simulink model "EngineDynamometer"  (R2025b)
settings: configuration reference "EngDynoVariable" (kept outside this file)
model workspace (MAT data in the model file):
  DynOperatingPts = timeseries
  DynOperatingPts.Name = 'Dynamic Operating Points'
  DynOperatingPts.DataInfo = tsdata.datametadata
  DynOperatingPts.DataInfo.Interpolation = tsdata.interpolation
  DynOperatingPts.DataInfo.Interpolation.Fhandle : function handle (value not decoded)
  DynOperatingPts.DataInfo.Interpolation.Name = 'linear'
  DynOperatingPts.TimeInfo = tsdata.timemetadata
  DynOperatingPts.TimeInfo.Length = 1281
  DynOperatingPts.TimeInfo.DuplicateTimes = 0
  DynOperatingPts.TimeInfo.Time_ = [0 0.001 7.75860549558 7.75960549558 8.75958684985 8.76058684985 10.7615495584 10.7625495584 11.7625309127 11.7635309127 13.7644936212 13.7654936212 ... (1281 elements, 1281x1)]
  DynOperatingPts.TimeInfo.Initialized = 1
  DynOperatingPts.QualityInfo = tsdata.qualmetadata
  DynOperatingPts.Data_ = [0 750 750 750 750 750 750 750 750 750 750 750 ... (2562 elements, 1281x2)]
undefined symbols (not defined in the file): CiDynoMaxTurboSpd, CiDynoSSSpdCmd, CiDynoSSTrqCmd, DynoResultsBlock, EnvAbsPrs, EnvAirTemp, EnvRair, ExhCamPhaseCmd, InjPw, IntkCamPhaseCmd, Line, PlntEngAfrStoich, PlntEngCps, PlntEngNCyl, PlntEngSinj, PlntEngVd, si, si0, SiDynoMaxTurboSpd, SiDynoOpenLoopEngSpdCmdPts, SiDynoOpenLoopExhCamPhsCmdPts, SiDynoOpenLoopIntCamPhsCmdPts, SiDynoOpenLoopLambdaCmdPts, SiDynoOpenLoopMaxMAP, SiDynoOpenLoopSpkDeltaCmdPts, SiDynoOpenLoopSteadyStateWaitLimit, SiDynoOpenLoopTpCmdPts, SiDynoOpenLoopWAPCmdPts, SiDynoSSSpdCmd, SiDynoSSTrqCmd, SiDynoSSWaitLim, SpkAdv, ThrPosPctCmd, WgAreaPctCmd
libraries: autolibutils x4, autolibpowerinfoutils x1, simulink x1
(part 1 of 3)
CloseFcn:
  | wkspvarnam = get_param(strcat(bdroot(gcb),'/Subsystem5'),'MbcTaskList');
  | clear(wkspvarnam)
  | clear wkspvarnam
settings Model: DataDictionary=VirtualDynoTemplate.sldd  ModifiedByFormat=The MathWorks, Inc.  SimulationMode=accelerator  PauseTimes=4395  NumberOfSteps=1000  SnapshotBufferSize=20  SnapshotInterval=1000  Creator=The MathWorks, Inc.  LastModifiedBy=The MathWorks, Inc.
settings ConfigSetRef: SourceName=EngDynoVariable

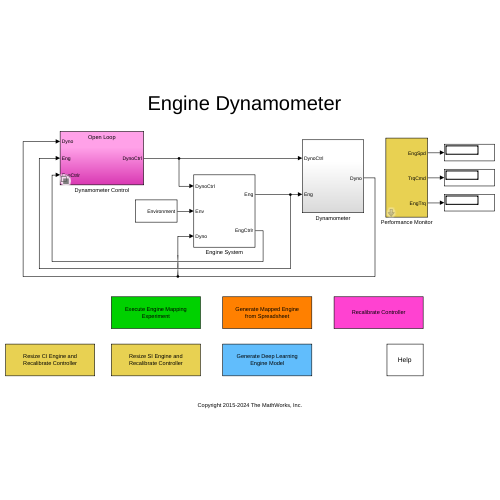
[thumbnail: Simulink's stored preview of the top-level diagram]
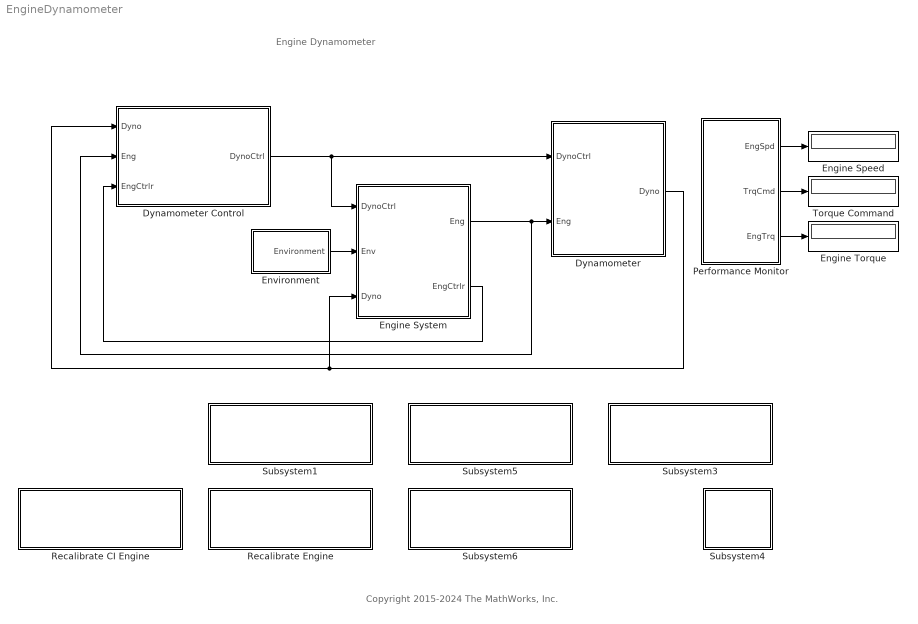
== system EngineDynamometer ==
  note: Engine Dynamometer
  note: Copyright 2015-2024 The MathWorks, Inc.
  Dynamometer : Subsystem
  Dynamometer Control : Subsystem  Variant=on  VariantControlMode=label  LabelModeActiveChoice=OpenLoop
  Engine Speed : Display
      settings: Decimation=100
  Engine System : Subsystem
      mask Display:
      | engplant = strcat(gcb,'/Engine Plant/Engine');
      | engvar = get_param(engplant,'ActiveVariant');
      | engvarp = strcat(engplant,'/',engvar);
      | istagged = false;
      | tagt = get_param(engvarp,'Tag');
      | if contains(engvar,'Mapped') && ~isempty(tagt)
      |     istagged = strcmp(tagt,'MappedEngCalByMBC');
      | end
      | ImageName = which('mbc_app_24.png');
      | if istagged
      |     if ~isempty(ImageName)
      |         IconImg = imread(ImageName,'png');
      |         MaskImg = 256*ones(150, 150,3);
      |         MaskImg = uint8(MaskImg);
      |         Xstart = 125;
      |         Ystart = 0;
      |         MaskImg((1:size(IconImg, 1))+Ystart, (1:size(IconImg, 2))+Xstart, 1:3) = IconImg;
      |         image(MaskImg);
      |     end
      |     disp('Mapped Engine\n Calibrated by\nMBC Toolbox')
      | end
  Engine Torque : Display
      settings: Decimation=100
  Environment : Subsystem
  Performance Monitor : Subsystem  StartFcn=DynoResultsBlock(gcb, 'StartFcn');  StopFcn=DynoResultsBlock(gcb, 'StopFcn');  mask(Performance Monitor){SteadyWsVarName=SteadyDynoSimOut, XVarPopup=Engine speed (rpm), YVarPopup=Torque command (N*m), ZVarPopup=Measured engine torque (N*m), DynWsVarName=DynamicDynoSimOut, DispAtEndCheckbox=on, UseSdiViewCheckbox=on, SdiRunName=Dynamometer Results, SdiViewFileName=DynoSDI_config.mldatx, ShowWaitbarCheckbox=on, NoPlot=si0}
      mask prompts: SteadyWsVarName "autoblks:autoblkDynoMask:wsVarName"; XVarPopup "autoblks:autoblkDynoMask:xAxisVar"; YVarPopup "autoblks:autoblkDynoMask:yAxisVar"; ZVarPopup "autoblks:autoblkDynoMask:zAxisVar"; DynWsVarName "autoblks:autoblkDynoMask:dynVarName"; DispAtEndCheckbox "autoblks:autoblkDynoMask:displayRes"; UseSdiViewCheckbox "autoblks:autoblkDynoMask:useSdiView"; SdiRunName "autoblks:autoblkDynoMask:sdiRunName"; SdiViewFileName "autoblks:autoblkDynoMask:sdiViewName"; ShowWaitbarCheckbox "autoblks:autoblkDynoMask:showWaitB"
      mask init:
      | DynoResultsBlock(gcb, 'Initialization');
      mask Help: helpview([docroot,'/toolbox/autoblks/helptargets.map'], 'siengine_dyno_refapp')
      mask TypeOptions XVarPopup: <EgrPct> | Air-fuel ratio | BSFC (g/(kW*hr)) | Compressor outlet temperature (C) | Compressor pressure ratio | EGR cooler outlet temperature (C) | EGR mass flow rate (g/s) | EGR valve area percent | EGR valve area percent command | Engine speed (rpm) | Engine speed command (rpm) | Estimated intake port mass flow rate (g/s) | Exhaust cam phase (degCrkRet) | Exhaust cam phase command (degCrkRet) | Exhaust manifold temperature (C) | Fuel mass flow rate (g/s) | Idle speed control torque command (N*m) | Injection pulse width (ms) | Intake cam phase (degCrkAdv) | Intake cam phase command (degCrkAdv) | Intake manifold pressure (kPa) | Intake manifold temperature (C) | Intake port mass flow rate (g/s) | Intercooler outlet temperature (C) | Load command | Measured engine torque (N*m) | Normalized air charge | Percent complete | Spark advance (degCrkAdv) | Steady state flag | Tailpipe CO emissions (g/s) | Tailpipe CO2 emissions (g/s) | Tailpipe HC emissions (g/s) | Tailpipe NOx emissions (g/s) | Throttle position percent | Throttle position percent command | Time (s) | Torque command (N*m) | Turbine outlet temperature (C) | Turbine pressure ratio | Turbocharger rack position | Turbocharger rack position command | Turbocharger shaft speed (rpm) | Wastegate area percent | Wastegate area percent command
      mask TypeOptions YVarPopup: None | <EgrPct> | Air-fuel ratio | BSFC (g/(kW*hr)) | Compressor outlet temperature (C) | Compressor pressure ratio | EGR cooler outlet temperature (C) | EGR mass flow rate (g/s) | EGR valve area percent | EGR valve area percent command | Engine speed (rpm) | Engine speed command (rpm) | Estimated intake port mass flow rate (g/s) | Exhaust cam phase (degCrkRet) | Exhaust cam phase command (degCrkRet) | Exhaust manifold temperature (C) | Fuel mass flow rate (g/s) | Idle speed control torque command (N*m) | Injection pulse width (ms) | Intake cam phase (degCrkAdv) | Intake cam phase command (degCrkAdv) | Intake manifold pressure (kPa) | Intake manifold temperature (C) | Intake port mass flow rate (g/s) | Intercooler outlet temperature (C) | Load command | Measured engine torque (N*m) | Normalized air charge | Percent complete | Spark advance (degCrkAdv) | Steady state flag | Tailpipe CO emissions (g/s) | Tailpipe CO2 emissions (g/s) | Tailpipe HC emissions (g/s) | Tailpipe NOx emissions (g/s) | Throttle position percent | Throttle position percent command | Time (s) | Torque command (N*m) | Turbine outlet temperature (C) | Turbine pressure ratio | Turbocharger rack position | Turbocharger rack position command | Turbocharger shaft speed (rpm) | Wastegate area percent | Wastegate area percent command
      mask TypeOptions ZVarPopup: None | <EgrPct> | Air-fuel ratio | BSFC (g/(kW*hr)) | Compressor outlet temperature (C) | Compressor pressure ratio | EGR cooler outlet temperature (C) | EGR mass flow rate (g/s) | EGR valve area percent | EGR valve area percent command | Engine speed (rpm) | Engine speed command (rpm) | Estimated intake port mass flow rate (g/s) | Exhaust cam phase (degCrkRet) | Exhaust cam phase command (degCrkRet) | Exhaust manifold temperature (C) | Fuel mass flow rate (g/s) | Idle speed control torque command (N*m) | Injection pulse width (ms) | Intake cam phase (degCrkAdv) | Intake cam phase command (degCrkAdv) | Intake manifold pressure (kPa) | Intake manifold temperature (C) | Intake port mass flow rate (g/s) | Intercooler outlet temperature (C) | Load command | Measured engine torque (N*m) | Normalized air charge | Percent complete | Spark advance (degCrkAdv) | Steady state flag | Tailpipe CO emissions (g/s) | Tailpipe CO2 emissions (g/s) | Tailpipe HC emissions (g/s) | Tailpipe NOx emissions (g/s) | Throttle position percent | Throttle position percent command | Time (s) | Torque command (N*m) | Turbine outlet temperature (C) | Turbine pressure ratio | Turbocharger rack position | Turbocharger rack position command | Turbocharger shaft speed (rpm) | Wastegate area percent | Wastegate area percent command
      mask DialogControl SteadyStateGroup Prompt: autoblks:autoblkDynoMask:steadySt
      mask DialogControl SteadyDesc Prompt: autoblks:autoblkDynoMask:steadyDesc
      mask DialogControl SteadyWsVarName Prompt: Steady state "To Workspace" variable name:
      mask DialogControl XVarPopup Prompt: X axis variable:
      mask DialogControl YVarPopup Prompt: Y axis variable:
      mask DialogControl ZVarPopup Prompt: Z axis variable:
      mask DialogControl PlotSteadyButton Prompt: autoblks:autoblkDynoMask:plotSS
      mask DialogControl PlotSteadyButton Callback: DynoResultsBlock(gcb, 'PlotSteadyButtonCallback');
      mask DialogControl DynamicGroup Prompt: autoblks:autoblkDynoMask:dynam
      mask DialogControl DynamicDesc Prompt: autoblks:autoblkDynoMask:plotDyn
      mask DialogControl DynWsVarName Prompt: Dynamic "To Workspace" variable name:
      mask DialogControl DispAtEndCheckbox Prompt: Display results at end of simulation
      mask DialogControl UseSdiViewCheckbox Prompt: Open Simulation Data Inspector view
      mask DialogControl SdiRunName Prompt: Simulation Data Inspector run name:
      mask DialogControl SdiViewFileName Prompt: Simulation Data Inspector view file name:
      mask DialogControl PlotDynamicButton Prompt: autoblks:autoblkDynoMask:plotDynButton
      mask DialogControl PlotDynamicButton Callback: DynoResultsBlock(gcb, 'PlotDynamicButtonCallback');
      mask DialogControl WaitbarGroup Prompt: autoblks:autoblkDynoMask:waitB
      mask DialogControl ShowWaitbarCheckbox Prompt: Show wait bar
  Recalibrate CI Engine : Subsystem  mask{EngReszSpecType=Displacement, EngReszMaxPwrDesIn=103.7766, EngReszDispDesIn=1.5, EngReszMaxPwrDes=109.307, EngReszNumCylDes=4, EngReszMaxPwr=103.7766, EngReszNumCyl=4, EngReszDisp=1.5, EngReszIdleSpd=500, EngReszMaxTqSpd=2750, EngReszMaxTq=273.6, EngReszBestFuelPwr=66, EngReszBestFuelSpd=2750, EngReszBestFuelTq=229.3, EngReszBestFuelBSFC=196.4, EngReszSpdMaxPwr=4000, EngReszTqMaxPwr=247.7, EngReszIntkManVol=2.86, EngReszExhManVol=0.7, EngReszMaxTurboSpd=237952.67, EngReszTurboRotInert=0.006, EngReszInjSlp=6.45}
      mask prompts: EngReszSpecType "Power or displacement"; EngReszMaxPwrDesIn "Desired maximum power [kW]:"; EngReszDispDesIn "Desired displacement [L]:"; EngReszMaxPwrDes "Desired maximum power [kW]:"; EngReszNumCylDes "Desired number of cylinders:"; EngReszMaxPwr "Maximum power [kW]:"; EngReszNumCyl "Number of cylinders:"; EngReszDisp "Engine displacement [L]:"; EngReszIdleSpd "Idle speed [rpm]:"; EngReszMaxTqSpd "Speed for maximum torque [rpm]:"; EngReszMaxTq "Maximum torque [Nm]:"; EngReszBestFuelPwr "Power for best fuel [kW]:"; EngReszBestFuelSpd "Speed for best fuel [rpm]:"; EngReszBestFuelTq "Torque for best fuel [Nm]:"; EngReszBestFuelBSFC "BSFC for best fuel [g/kWh]:"; EngReszSpdMaxPwr "Speed for maximum power [rpm]:"; EngReszTqMaxPwr "Torque for maximum power [Nm]:"; EngReszIntkManVol "Intake manifold volume [L]:"; EngReszExhManVol "Exhaust manifold volume [L]:"; EngReszMaxTurboSpd "Maximum turbo speed [rpm]:"; EngReszTurboRotInert "Turbo rotor inertia [kg*m^2]:"; EngReszInjSlp "Fuel injector slope [mg/ms]:"
      mask help: Resize engine plant and re-calibrate engine controller based on desired maximum power level or displacement, and number of cylinders
      settings: OpenFcn=|
      | block=[bdroot '/Recalibrate CI Engine'];
      | 
      | modelStatus = get_param(bdroot,'SimulationStatus');
      | 
      | if ~bdIsLibrary(bdroot) && strcmp(modelStatus,'stopped')
      |    autoicon('autolibciengresize',block,'open');
      |    open_system(block,'mask');
      | elseif ~bdIsLibrary(bdroot) && ~strcmp(modelStatus,'stopped')
      | else
      | end
      | 
      | clear modelStatus;
      | clear block;
      mask Help: eval('autoblkshelp(''pt_ci_resize'')');
      mask TypeOptions EngReszSpecType: Power | Displacement
      mask Callback EngReszSpecType: autoicon('autolibciengresize',gcb,'resizebasis');
      mask DialogControl DescGroupVar Prompt: Resize engine and recalibrate controller
      mask DialogControl DescTextVar Prompt: Resize engine plant and re-calibrate engine controller based on desired maximum power level or displacement, and number of cylinders
      mask DialogControl ResizeEngButton Prompt: Resize Engine
      mask DialogControl ResizeEngButton Callback: autoicon('autolibciengresize',gcb,'resize');
      mask DialogControl CurrEngDesign Prompt: Current Engine Design
      mask Display: disp(getString(message('autoblks:autoblkDynoMask:resizeCiLabel')))
  Recalibrate Engine : Subsystem  mask(Engine resize and recalibrate tool){EngReszSpecType=Displacement, EngReszMaxPwrDesIn=115.0917, EngReszDispDesIn=1.5, EngReszMaxPwrDes=115.0917, EngReszNumCylDes=4, EngReszArchEngine=Line, EngReszTurb=on, EngReszEgr=on, Thr2=off, TrqSpec=off, EngReszDesMaxTq=228, TrqSpdSpec=off, EngReszReqMaxTqSpd=2571, EngReszMaxPwr=115.0917, EngReszDisp=1.5, EngReszNumCyl=4, EngReszIdleSpd=750, EngReszMaxTqSpd=2571, EngReszMaxTq=228, EngReszBestFuelPwr=41.1, EngReszBestFuelSpd=2571, EngReszBestFuelTq=152.7, EngReszBestFuelBSFC=225.9, EngReszSpdMaxPwr=5000, EngReszTqMaxPwr=219.8, EngReszThrDiam=50, EngReszIntkManVol=2.86, EngReszExhManVol=1.6, EngReszCompOutVol=2.6, EngReszMaxTurboSpd=232000, EngReszTurboRotInert=0.016, EngReszInjSlp=6.45, EngCurrArch=Line, EngCurrTurb=on, EngCurrEGR=on, EngCurrThr2=off, EngCurrMaxTq=0, EngCurrMaxTqSpd=0}
      mask prompts: EngReszSpecType "autoblks:autoblkDynoMask:powerOrDispl"; EngReszMaxPwrDesIn "autoblks:autoblkDynoMask:desMaxPower"; EngReszDispDesIn "autoblks:autoblkDynoMask:desMaxDispl"; EngReszMaxPwrDes "autoblks:autoblkDynoMask:desMaxPower"; EngReszNumCylDes "autoblks:autoblkDynoMask:desNCyls"; EngReszArchEngine "autoblks:autoblkDynoMask:engArch"; EngReszTurb "autoblks:autoblkDynoMask:turbo"; EngReszEgr "autoblks:autoblkDynoMask:egr"; Thr2 "autoblks:autoblkDynoMask:twinInt"; TrqSpec "autoblks:autoblkDynoMask:maxTrq"; EngReszDesMaxTq "autoblks:autoblkDynoMask:desTrq"; TrqSpdSpec "autoblks:autoblkDynoMask:spdTrq"; EngReszReqMaxTqSpd "autoblks:autoblkDynoMask:desSpd"; EngReszMaxPwr "autoblks:autoblkDynoMask:maxPwr"; EngReszDisp "autoblks:autoblkDynoMask:engDispl"; EngReszNumCyl "autoblks:autoblkDynoMask:nCyls"; EngReszIdleSpd "autoblks:autoblkDynoMask:idleSpd"; EngReszMaxTqSpd "autoblks:autoblkDynoMask:trqSpd"; EngReszMaxTq "autoblks:autoblkDynoMask:actTrq"; EngReszBestFuelPwr "autoblks:autoblkDynoMask:bestFuel"; EngReszBestFuelSpd "autoblks:autoblkDynoMask:bestSpd"; EngReszBestFuelTq "autoblks:autoblkDynoMask:bestTrq"; EngReszBestFuelBSFC "autoblks:autoblkDynoMask:bestBSFC"; EngReszSpdMaxPwr "autoblks:autoblkDynoMask:maxPwrSpd"; EngReszTqMaxPwr "autoblks:autoblkDynoMask:trqPwr"; EngReszThrDiam "autoblks:autoblkDynoMask:thrDia"; EngReszIntkManVol "autoblks:autoblkDynoMask:intVol"; EngReszExhManVol "autoblks:autoblkDynoMask:exhVol"; EngReszCompOutVol "autoblks:autoblkDynoMask:cmpVol"; EngReszMaxTurboSpd "autoblks:autoblkDynoMask:turboSpd"; EngReszTurboRotInert "autoblks:autoblkDynoMask:tInertia"; EngReszInjSlp "autoblks:autoblkDynoMask:injFlow"; EngCurrArch "autoblks:autoblkDynoMask:engArch"; EngCurrTurb "autoblks:autoblkDynoMask:turbo"; EngCurrEGR "autoblks:autoblkDynoMask:egr"; EngCurrThr2 "autoblks:autoblkDynoMask:twinInt"; EngCurrMaxTq "autoblks:autoblkDynoMask:desTrq"; EngCurrMaxTqSpd "autoblks:autoblkDynoMask:desSpd"
      mask help: autoblks:autoblkDynoMask:descText
      mask init:
      | autoicon('autolibsiengresize',gcb,'updateEng');
      settings: OpenFcn=|
      | block=[bdroot '/Recalibrate Engine'];
      | 
      | modelStatus = get_param(bdroot,'SimulationStatus');
      | 
      | if ~bdIsLibrary(bdroot) && strcmp(modelStatus,'stopped')
      |    autoicon('autolibsiengresize',block,'open');
      |    open_system(block,'mask');
      | end
      | 
      | clear modelStatus;
      | clear block;
      mask Help: eval('autoblkshelp(''pt_si_resize'')');
      mask TypeOptions EngReszSpecType: autoblks:autoblkDynoMask:pOpt | autoblks:autoblkDynoMask:dOpt
      mask Callback EngReszSpecType:
      | if autoblkschecksimstopped(gcb)
      |     autoicon('autolibsiengresize',gcb,'resizebasis');
      |     maskObj = Simulink.Mask.get(gcb);
      |     if strcmp(maskObj.getParameter('EngReszSpecType').Value,getString(message('autoblks:autoblkDynoMask:pOpt')))
      |         maskObj.getParameter('TrqSpec').set('Visible','off');
      |         maskObj.getParameter('TrqSpdSpec').set('Visible','off');
      |         maskObj.getParameter('EngReszDesMaxTq').set('Visible','off');
      |         maskObj.getParameter('EngReszReqMaxTqSpd').set('Visible','off');
      |     else
      |         maskObj.getParameter('TrqSpec').set('Visible','on');
      |         maskObj.getParameter('TrqSpdSpec').set('Visible','on');
      |         if strcmp(maskObj.getParameter('TrqSpec').Value,'on')
      |             maskObj.getParameter('EngReszDesMaxTq').set('Visible','on');
      |         end
      |         if strcmp(maskObj.getParameter('TrqSpdSpec').Value,'on')
      |             maskObj.getParameter('EngReszReqMaxTqSpd').set('Visible','on');
      |         end
      |     end
      | end
      mask TypeOptions EngReszArchEngine: autoblks:autoblkDynoMask:iOpt | autoblks:autoblkDynoMask:vOpt
      mask Callback EngReszArchEngine:
      | if autoblkschecksimstopped(gcb)
      |     maskObj = Simulink.Mask.get(gcb);
      |     thr2box = maskObj.getParameter('Thr2');
      |     if strcmp(maskObj.getParameter('EngReszArchEngine').Value,getString(message('autoblks:autoblkDynoMask:vOpt'))) && ...
      |             strcmp(maskObj.getParameter('EngReszTurb').Value,'on')
      |         thr2box.set('Visible','on');
      |     else
      |         thr2box.set('Visible','off');
      |     end
      | end
      mask Callback EngReszTurb:
      | if autoblkschecksimstopped(gcb)
      |     maskObj = Simulink.Mask.get(gcb);
      |     thr2box = maskObj.getParameter('Thr2');
      |     if strcmp(maskObj.getParameter('EngReszTurb').Value,'on')
      |         maskObj.getParameter('EngReszCompOutVol').set('Visible','on');
      |         maskObj.getParameter('EngReszMaxTurboSpd').set('Visible','on');
      |         maskObj.getParameter('EngReszTurboRotInert').set('Visible','on');
      |         if strcmp(maskObj.getParameter('EngReszArchEngine').Value,getString(message('autoblks:autoblkDynoMask:vOpt'))) && ...
      |                 strcmp(thr2box.Visible,'off')
      |             thr2box.set('Visible','on');
      |         end
      |     else
      |         maskObj.getParameter('EngReszCompOutVol').set('Visible','off');
      |         maskObj.getParameter('EngReszMaxTurboSpd').set('Visible','off');
      |         maskObj.getParameter('EngReszTurboRotInert').set('Visible','off');
      |         if strcmp(maskObj.getParameter('EngReszArchEngine').Value,getString(message('autoblks:autoblkDynoMask:vOpt'))) && ...
      |                 strcmp(thr2box.Visible,'on')
      |             thr2box.set('Visible','off');
      |         end
      |     end
      | end
      mask Callback TrqSpec:
      | if autoblkschecksimstopped(gcb)
      |     autoicon('autolibsiengresize',gcb,'defTrq'); % Update with default calculated value
      |     maskObj = Simulink.Mask.get(gcb);
      |     maskTrq = get_param(gcb,'EngReszDesMaxTq'); % Need to get the value set from autoblkssiengresize in order to update
      |     if strcmp(maskObj.getParameter('TrqSpec').Value,'on')
      |         maskObj.getParameter('EngReszDesMaxTq').set('Visible','on');
      |         set_param(gcb,'EngReszDesMaxTq',maskTrq); % Need to set updated value in order to update
      |     else
      |         maskObj.getParameter('EngReszDesMaxTq').set('Visible','off');
      |     end
      | end
      mask Callback TrqSpdSpec:
      | if autoblkschecksimstopped(gcb)
      |     autoicon('autolibsiengresize',gcb,'defSpd'); % Populate with calculated default value
      |     maskObj = Simulink.Mask.get(gcb);
      |     maskSpd = get_param(gcb,'EngReszReqMaxTqSpd'); % Need to get the value set from autoblkssiengresize in order to update
      |     if strcmp(maskObj.getParameter('TrqSpdSpec').Value,'on')
      |         maskObj.getParameter('EngReszReqMaxTqSpd').set('Visible','on');
      |         set_param(gcb,'EngReszReqMaxTqSpd',maskSpd); % Need to set updated value in order to update
      |     else
      |         maskObj.getParameter('EngReszReqMaxTqSpd').set('Visible','off');
      |     end
      | end
      mask DialogControl Container4 Prompt: autoblks:autoblkDynoMask:design
      mask DialogControl EngReszSpecType Prompt: Resize option
      mask DialogControl EngReszMaxPwrDesIn Prompt: Desired maximum power, EngReszMaxPwrDes [kW]:
      mask DialogControl EngReszDispDesIn Prompt: Desired displacement, EngReszDispDesIn [L]:
      mask DialogControl EngReszMaxPwrDes Prompt: Desired maximum power, EngReszMaxPwrDes [kW]:
      mask DialogControl EngReszNumCylDes Prompt: Desired number of cylinders, EngReszNumCylDes [-]:
      mask DialogControl EngReszArchEngine Prompt: Architecture
      mask DialogControl EngReszTurb Prompt: Turbocharger
      mask DialogControl EngReszEgr Prompt: EGR
      mask DialogControl Thr2 Prompt: Twin Intake
      mask DialogControl TrqSpec Prompt: Specify maximum torque
      mask DialogControl EngReszDesMaxTq Prompt: EngReszDesMaxTq [Nm]:
      mask DialogControl TrqSpdSpec Prompt: Specify speed at maximum torque
      mask DialogControl EngReszReqMaxTqSpd Prompt: EngReszReqMaxTqSpd [rpm]:
      mask DialogControl ResizeEngButton Prompt: autoblks:autoblkDynoMask:resizeButton
      mask DialogControl ResizeEngButton Callback: autoicon('autolibsiengresize',gcb,'resize');
      mask DialogControl Container6 Prompt: autoblks:autoblkDynoMask:perfSpecs
      mask DialogControl CurrEngDesign Prompt: autoblks:autoblkDynoMask:currEng
      mask DialogControl EngReszMaxPwr Prompt: Maximum power [kW]:
      mask DialogControl EngReszDisp Prompt: Engine displacement [L]:
      mask DialogControl EngReszNumCyl Prompt: Number of cylinders:
      mask DialogControl EngReszIdleSpd Prompt: Idle speed [rpm]:
      mask DialogControl EngReszMaxTqSpd Prompt: Speed for maximum torque [rpm]:
      mask DialogControl EngReszMaxTq Prompt: Maximum torque [Nm]:
      mask DialogControl EngReszBestFuelPwr Prompt: Power for best fuel [kW]:
      mask DialogControl EngReszBestFuelSpd Prompt: Speed for best fuel [rpm]:
      mask DialogControl EngReszBestFuelTq Prompt: Torque for best fuel [Nm]:
      mask DialogControl EngReszBestFuelBSFC Prompt: BSFC for best fuel [g/kWh]:
      mask DialogControl EngReszSpdMaxPwr Prompt: Speed for maximum power [rpm]:
      mask DialogControl EngReszTqMaxPwr Prompt: Torque for maximum power [Nm]:
      mask DialogControl EngReszThrDiam Prompt: Throttle bore diameter [mm]:
      mask DialogControl EngReszIntkManVol Prompt: Intake manifold volume [L]:
      mask DialogControl EngReszExhManVol Prompt: Exhaust manifold volume [L]:
      mask DialogControl EngReszCompOutVol Prompt: Compressor out volume [L]:
      mask DialogControl EngReszMaxTurboSpd Prompt: Maximum turbo speed [rpm]:
      mask DialogControl EngReszTurboRotInert Prompt: Turbo rotor inertia [kg*m^2]:
      mask DialogControl EngReszInjSlp Prompt: Fuel injector slope [mg/ms]:
      mask DialogControl EngCurrArch Prompt: Architecture
      mask DialogControl EngCurrTurb Prompt: Turbocharger
      mask DialogControl EngCurrEGR Prompt: EGR
      mask DialogControl EngCurrThr2 Prompt: Twin Intake
      mask DialogControl EngCurrMaxTq Prompt: EngReszDesMaxTq [Nm]:
      mask DialogControl EngCurrMaxTqSpd Prompt: EngReszReqMaxTqSpd [rpm]:
      mask Display: disp(getString(message('autoblks:autoblkDynoMask:resizeSiLabel')))
  Subsystem1 : Subsystem
      settings: OpenFcn=DynamometerStart(gcb, 'SteadyState')
      mask Display: disp(getString(message('autoblks:autoblkDynoMask:engMapLabel')))
  Subsystem3 : Subsystem  mask{NoMsk=0}
      settings: OpenFcn=|
      | engblk=[bdroot,'/Engine System/Engine Plant/Engine'];
      | engvar=get_param(engblk,'ActiveVariant');
      | if strcmp(engvar,'CI Engine') || strcmp(engvar,'CI Mapped Engine')
      |   RecalibrateCIController(gcb, 'OpenFcn')
      | else
      |   RecalibrateSIController(gcb, 'OpenFcn')
      | end
      | clear engblk engvar
      mask Display: disp(getString(message('autoblks:autoblkDynoMask:recalibLabel')))
  Subsystem4 : Subsystem  mask{SiOrCi=si}
      settings: OpenFcn=|
      | if strcmp(get_param(gcb, 'SiOrCi'),'sih2')
      |   helpview([docroot,'/toolbox/autoblks/helptargets.map'], 'sih2engine_dyno_refapp')
      | elseif strcmp(get_param(gcb, 'SiOrCi'),'ci')
      |   helpview([docroot,'/toolbox/autoblks/helptargets.map'], 'ciengine_dyno_refapp')
      | else
      |   helpview([docroot,'/toolbox/autoblks/helptargets.map'], 'siengine_dyno_refapp')
      | end
      mask Display: disp(getString(message('autoblks:autoblkDynoMask:helpLabel')))
  Subsystem5 : Subsystem  LoadFcn=[~]=GenerateMappedEngineCalibrations(gcb, 'CheckMBCLicense');  mask(Create Mapped Engine from Spreadsheet){SpreadsheetFileName=SiEngineData.xlsx, MappedEngMdlRefName=SiMappedEngine, MbcTaskList=mbctasklist}
      mask prompts: SpreadsheetFileName "autoblks:autoblkDynoMask:mapSheetFile"; MappedEngMdlRefName "autoblks:autoblkDynoMask:mappedEng"; MbcTaskList "MBC Task List"
      mask help: autoblks:autoblkDynoMask:descSheet
      mask init:
      | GenerateMappedEngineCalibrations(gcb, 'Init');
      settings: OpenFcn=|
      | [~]=GenerateMappedEngineCalibrations(gcb, 'EnableCalToolButton');
      | open_system(gcb, 'mask')
      mask Help: helpview([docroot,'/toolbox/autoblks/helptargets.map'], 'siengine_dyno_mapped')
      mask DialogControl DescTextVar Prompt: autoblks:autoblkDynoMask:descSheet
      mask DialogControl MBCHyperlink Prompt: autoblks:autoblkDynoMask:reqOpt
      mask DialogControl MBCHyperlink Callback: helpview([docroot,'/toolbox/mbc/helptargets.map'], 'mbc_landing_page')
      mask DialogControl Container3 Prompt: autoblks:autoblkDynoMask:step1
      mask DialogControl SpreadsheetFileName Prompt: Spreadsheet file:
      mask DialogControl SpreadsheetFileNameSelect Prompt: autoblks:autoblkDynoMask:ellipsis
      mask DialogControl SpreadsheetFileNameSelect Callback: GenerateMappedEngineCalibrations(gcb, 'SpreadsheetFileNameSelect');
      mask DialogControl GenMappedEngCalButton Prompt: autoblks:autoblkDynoMask:engCal
      mask DialogControl GenMappedEngCalButton Callback: GenerateMappedEngineCalibrations(gcb, 'GenMappedEngCalButton');
      mask DialogControl OpenCalToolButton Prompt: autoblks:autoblkDynoMask:openCal
      mask DialogControl OpenCalToolButton Callback: GenerateMappedEngineCalibrations(gcb, 'OpenMBCFiles');
      mask DialogControl MappedEngMdlRefName Prompt: Mapped engine model reference name
      mask Display: disp(getString(message('autoblks:autoblkDynoMask:mapSpreadLabel')))
  Subsystem6 : Subsystem
      settings: OpenFcn=[~,~,~,~,~]=FitSiEngineDL(bdroot(gcb));
      mask Display: disp(getString(message('autoblks:autoblkDynoMask:genDLengLabel')))
  Torque Command : Display
      settings: Decimation=100
  wires:
  Engine System/2(EngCtrlr) -> Dynamometer Control/3(EngCtrlr)
  Dynamometer Control/1(DynoCtrl) -> Dynamometer/1(DynoCtrl), Engine System/1(DynoCtrl)
  Dynamometer/1(Dyno) -> Dynamometer Control/1(Dyno), Engine System/3(Dyno)
  Engine System/1(Eng) -> Dynamometer Control/2(Eng), Dynamometer/2(Eng)
  Environment/1(Environment) -> Engine System/2(Env)
  Performance Monitor/3(EngTrq) -> Engine Torque/1
  Performance Monitor/1(EngSpd) -> Engine Speed/1
  Performance Monitor/2(TrqCmd) -> Torque Command/1

== system EngineDynamometer/Dynamometer ==
  DynoCtrl : Inport
  Eng : Inport  Port=2
  Bus Creator : BusCreator  Inputs=2
  Bus Selector : BusSelector  OutputSignals=EngPlnt.EngTrq,EngPlnt.EngSpdOut
  Dynamometer Motor Controller : Subsystem
  Dynamometer Plant : Subsystem
  Bus Element Out1 : Outport  PortName=Dyno  Element=DynoPlnt
  Bus Element Out : Outport  PortName=Dyno  Element=DynoCtrl
  tag scope: DynoResults=global
  wires:
  Bus Creator/1 -> [DynoResults]
  Eng/1 -> Bus Selector/1, Dynamometer Plant/1(Eng), Dynamometer Motor Controller/1(EngPlnt)
  Dynamometer Plant/1(DynoPlnt) -> [DynoPlnt], Bus Element Out1/1, Dynamometer Motor Controller/3(DynoPlnt)
  Dynamometer Motor Controller/1(DynoMotorCtrl) -> Dynamometer Plant/4(DynoCtrl)
  [DynoPlnt] -> Bus Creator/2  "DynoPlnt"
  [DynoCtrl] -> Bus Creator/1  "DynoCtrl"
  DynoCtrl/1 -> Bus Element Out/1, [DynoCtrl], Dynamometer Motor Controller/2(DynoCtrl)
  Bus Selector/1 -> Dynamometer Plant/2(EngTrq)  "<EngTrq>"
  Bus Selector/2 -> Dynamometer Plant/3("EngSpd ")  "<EngSpdOut>"

== system EngineDynamometer/Dynamometer Control ==
  Dyno : Inport
  Eng : Inport  Port=2
  EngCtrlr : Inport  Port=3
  Calibrate Throttle and Wastegate : Subsystem  VariantControl=CalThrWg
  Calibration Controller : Subsystem  VariantControl=CalCtrl
  Dynamic : Subsystem  VariantControl=Dynamic
  Open Loop : Subsystem  VariantControl=OpenLoop
  Steady State : Subsystem  VariantControl=SteadyState
  DynoCtrl : Outport  VectorParamsAs1DForOutWhenUnconnected=off

== system EngineDynamometer/Engine System ==
  DynoCtrl : Inport
  Env : Inport  Port=2
  Dyno : Inport  Port=3
  Bus Creator : BusCreator  Inputs=4
  Dynamometer Engine Control : Subsystem
  Engine Controller : Subsystem
  Engine Plant : Subsystem
  Eng : Outport  VectorParamsAs1DForOutWhenUnconnected=off
  EngCtrlr : Outport  Port=2  VectorParamsAs1DForOutWhenUnconnected=off
  tag scope: EngSysResults=global
  wires:
  Dynamometer Engine Control/1(Ctrl) -> Engine Plant/2(Ctrl), [EngCtrl]
  Dyno/1 -> Engine Plant/3(Dyno), Dynamometer Engine Control/1(Dyno)
  Env/1 -> Engine Controller/1(Env), [Env], Engine Plant/1(Env)
  Bus Creator/1 -> Eng/1, [EngSysResults]
  [EngPlnt] -> Bus Creator/2  "EngPlnt"
  [EngCtrl] -> Bus Creator/1  "EngCtrl"
  Engine Controller/1(EngCtrlrOutput) -> EngCtrlr/1, [EngCtrlrOutput]
  [EngCtrlrOutput] -> Bus Creator/3  "EngCtrlrOutput"
  DynoCtrl/1 -> Engine Controller/2(Dyno)
  Engine Plant/1(EngFdbk) -> Engine Controller/3(EngPlnt), [EngPlnt]
  [Env] -> Bus Creator/4  "Env"

== system EngineDynamometer/Environment ==
  Bus Creator : BusCreator  Inputs=4
  Bus Creator3 : BusCreator  Inputs=3
  Bus Creator4 : BusCreator  Inputs=2
  Bus Creator5 : BusCreator  Inputs=2
  Constant : Constant  Value=1.*ones(4,1)
  Constant1 : Constant  Value=1.*ones(4,1)
  Constant{2..5} (4 alike) : Constant  Value=0
  Constant6 : Constant  Value=EnvAirTemp+7
  Constant7 : Constant  Value=EnvAbsPrs
  Environment : Outport  VectorParamsAs1DForOutWhenUnconnected=off
  wires:
  Constant/1 -> Bus Creator5/1  "lam_mu_x"
  Constant1/1 -> Bus Creator5/2  "lam_mu_y"
  Bus Creator5/1 -> Bus Creator4/2  "Ground_mu"
  Bus Creator4/1 -> Bus Creator/3  "Ground"
  Bus Creator3/1 -> Bus Creator/4  "Wind"
  Constant3/1 -> Bus Creator3/1  "wind_x"
  Constant4/1 -> Bus Creator3/2  "wind_y"
  Constant5/1 -> Bus Creator3/3  "wind_z"
  Constant6/1 -> Bus Creator/1  "AmbTemp"
  Constant2/1 -> Bus Creator4/1  "Grade"
  Bus Creator/1 -> Environment/1  "Environment"
  Constant7/1 -> Bus Creator/2  "BaroPress"

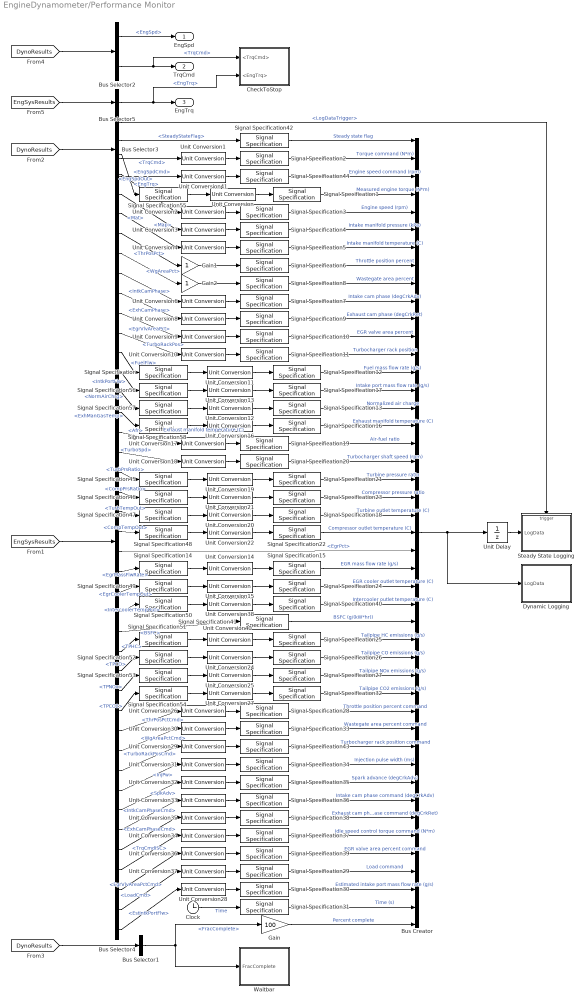
== system EngineDynamometer/Performance Monitor ==
  Bus Creator : BusCreator  Inputs=45
  Bus Selector1 : BusSelector  OutputSignals=DynoCtrl.DynoCtrl.FracComplete
  Bus Selector2 : BusSelector  OutputSignals=DynoPlnt.EngSpd,DynoCtrl.DynoCtrl.TrqCmd
  Bus Selector3 : BusSelector  OutputSignals=DynoCtrl.DynoCtrl.LogDataTrigger,DynoCtrl.DynoCtrl.SteadyStateFlag,DynoCtrl.DynoCtrl.TrqCmd,DynoCtrl.DynoCtrl.EngSpdCmd
  Bus Selector4 : BusSelector  OutputSignals=EngPlnt.EngTrq,EngPlnt.EngSpdOut,EngPlnt.Map,EngPlnt.Mat,EngPlnt.ThrPosPct,EngPlnt.WgAreaPct,EngPlnt.IntkCamPhase,EngPlnt.ExhCamPhase,EngPlnt.EgrVlvAreaPct,EngPlnt.TurboRackPos,EngPlnt.FuelFlw,EngPlnt.IntkPortFlw,EngPlnt.NormAirChrg,EngPlnt.ExhManGasTemp,EngPlnt.Afr,EngPlnt.TurboSpd,EngPlnt.TurbPrsRatio,EngPlnt.CompPrsRatio,EngPlnt.TurbTempOut,EngPlnt.CompTempOut,EngPlnt.EgrPct,EngPlnt.EgrMassFlwRate,EngPlnt.EgrCoolerTempOut,EngPlnt.IntercoolerTempOut,EngPlnt.BSFC,EngPlnt.TPHC,EngPlnt.TPCO,EngPlnt.TPNOx,EngPlnt.TPCO2,EngCtrl.ThrPosPctCmd,EngCtrl.WgAreaPctCmd,EngCtrl.TurboRackPosCmd,EngCtrl.InjPw,EngCtrl.SpkAdv,EngCtrl.IntkCamPhaseCmd,EngCtrl.ExhCamPhaseCmd,EngCtrl.TrqCmdISC,EngCtrl.EgrVlvAreaPctCmd,EngCtrl.LoadCmd,EngCtrl.EstIntkPortFlw
  Bus Selector5 : BusSelector  OutputSignals=EngPlnt.EngTrq
  CheckToStop : Subsystem
  Clock : Clock
  Dynamic Logging : Subsystem
  Gain : Gain  Gain=100
  Gain1 : Gain
  Gain2 : Gain
  Signal Specification{,14,51..54,56} (7 alike) : SignalSpecification  Unit=kg/s
  Signal Specification{1..2,37,55} (4 alike) : SignalSpecification  Unit=N*m
  Signal Specification{6,8,10,28,33,39} (6 alike) : SignalSpecification  Unit=%
  Signal Specification{11,13,19,21,23,29,42..43,45..46,57} (11 alike) : SignalSpecification  Unit=1
  Signal Specification{12,15,17,25..27,30,32} (8 alike) : SignalSpecification  Unit=g/s
  Signal Specification{5,16,18,22,24,40} (6 alike) : SignalSpecification  Unit=°C
  Signal Specification20 : SignalSpecification  Unit=rpm
  Signal Specification3 : SignalSpecification  Unit=rpm
  Signal Specification31 : SignalSpecification  Unit=s
  Signal Specification34 : SignalSpecification  Unit=ms
  Signal Specification{7,9,35..36,38} (5 alike) : SignalSpecification  Unit=deg
  Signal Specification4 : SignalSpecification  Unit=kPa
  Signal Specification41 : SignalSpecification  Unit=g/(kW*hr)
  Signal Specification44 : SignalSpecification  Unit=rpm
  Signal Specification{47..50,58} (5 alike) : SignalSpecification  Unit=K
  Steady State Logging : Subsystem
  Unit Conversion{,1..4,6,8..22,24..38,40..41} (38 alike) : UnitConversion
  Unit Delay : UnitDelay  SampleTime=-1  HasFrameUpgradeWarning=on
  Waitbar : Subsystem  StartFcn=""
  EngSpd : Outport  VectorParamsAs1DForOutWhenUnconnected=off
  TrqCmd : Outport  Port=2  VectorParamsAs1DForOutWhenUnconnected=off
  EngTrq : Outport  Port=3  VectorParamsAs1DForOutWhenUnconnected=off
  wires:
  Gain/1 -> Bus Creator/45  "Percent complete"
  Signal Specification9/1 -> Bus Creator/11  "Exhaust cam phase (degCrkRet)"
  Signal Specification8/1 -> Bus Creator/9  "Wastegate area percent"
  Signal Specification7/1 -> Bus Creator/10  "Intake cam phase (degCrkAdv)"
  Signal Specification6/1 -> Bus Creator/8  "Throttle position percent"
  Signal Specification5/1 -> Bus Creator/7  "Intake manifold temperature (C)"
  Signal Specification43/1 -> Bus Creator/35  "Turbocharger rack position command"
  Signal Specification41/1 -> Bus Creator/28  "BSFC (g/(kW*hr))"
  Signal Specification40/1 -> Bus Creator/27  "Intercooler outlet temperature (C)"
  Signal Specification4/1 -> Bus Creator/6  "Intake manifold pressure (kPa)"
  Signal Specification39/1 -> Bus Creator/41  "EGR valve area percent command"
  Signal Specification38/1 -> Bus Creator/39  "Exhaust cam phase command (degCrkRet)"
  Signal Specification37/1 -> Bus Creator/40  "Idle speed control torque command (N*m)"
  Signal Specification36/1 -> Bus Creator/38  "Intake cam phase command (degCrkAdv)"
  Signal Specification35/1 -> Bus Creator/37  "Spark advance (degCrkAdv)"
  Signal Specification34/1 -> Bus Creator/36  "Injection pulse width (ms)"
  Signal Specification33/1 -> Bus Creator/34  "Wastegate area percent command"
  Signal Specification32/1 -> Bus Creator/32  "Tailpipe CO2 emissions (g/s)"
  Signal Specification31/1 -> Bus Creator/44  "Time (s)"
  Signal Specification30/1 -> Bus Creator/43  "Estimated intake port mass flow rate (g/s)"
  Signal Specification3/1 -> Bus Creator/5  "Engine speed (rpm)"
  Signal Specification29/1 -> Bus Creator/42  "Load command"
  Signal Specification28/1 -> Bus Creator/33  "Throttle position percent command"
  Signal Specification27/1 -> Bus Creator/31  "Tailpipe NOx emissions (g/s)"
  Signal Specification26/1 -> Bus Creator/30  "Tailpipe CO emissions (g/s)"
  Signal Specification25/1 -> Bus Creator/29  "Tailpipe HC emissions (g/s)"
  Signal Specification24/1 -> Bus Creator/26  "EGR cooler outlet temperature (C)"
  Signal Specification23/1 -> Bus Creator/21  "Compressor pressure ratio"
  Signal Specification22/1 -> Bus Creator/23  "Compressor outlet temperature (C)"
  Signal Specification21/1 -> Bus Creator/20  "Turbine pressure ratio"
  Signal Specification20/1 -> Bus Creator/19  "Turbocharger shaft speed (rpm)"
  Signal Specification19/1 -> Bus Creator/18  "Air-fuel ratio"
  Signal Specification18/1 -> Bus Creator/22  "Turbine outlet temperature (C)"
  Signal Specification17/1 -> Bus Creator/15  "Intake port mass flow rate (g/s)"
  Signal Specification16/1 -> Bus Creator/17  "Exhaust manifold temperature (C)"
  Signal Specification15/1 -> Bus Creator/25  "EGR mass flow rate (g/s)"
  Signal Specification13/1 -> Bus Creator/16  "Normalized air charge"
  Signal Specification12/1 -> Bus Creator/14  "Fuel mass flow rate (g/s)"
  Signal Specification11/1 -> Bus Creator/13  "Turbocharger rack position"
  Signal Specification10/1 -> Bus Creator/12  "EGR valve area percent"
  Signal Specification1/1 -> Bus Creator/4  "Measured engine torque (N*m)"
  Signal Specification44/1 -> Bus Creator/3  "Engine speed command (rpm)"
  Bus Selector3/4 -> Unit Conversion41/1  "<EngSpdCmd>"
  Unit Conversion41/1 -> Signal Specification44/1
  Signal Specification2/1 -> Bus Creator/2  "Torque command (N*m)"
  Bus Selector5/1 -> CheckToStop/2(<EngTrq>), EngTrq/1  "<EngTrq>"
  [EngSysResults] -> Bus Selector5/1
  Bus Selector2/2 -> CheckToStop/1(<TrqCmd>), TrqCmd/1  "<TrqCmd>"
  Bus Selector2/1 -> EngSpd/1  "<EngSpd>"
  [DynoResults] -> Bus Selector2/1
  [DynoResults] -> Bus Selector1/1
  Bus Selector1/1 -> Gain/1, Waitbar/1(FracComplete)  "<FracComplete>"
  Signal Specification42/1 -> Bus Creator/1  "Steady state flag"
  Bus Selector4/40 -> Unit Conversion28/1  "<EstIntkPortFlw>"
  Bus Selector4/39 -> Unit Conversion37/1  "<LoadCmd>"
  Bus Selector4/38 -> Unit Conversion36/1  "<EgrVlvAreaPctCmd>"
  Bus Selector4/37 -> Unit Conversion34/1  "<TrqCmdISC>"
  Bus Selector4/36 -> Unit Conversion35/1  "<ExhCamPhaseCmd>"
  Bus Selector4/35 -> Unit Conversion33/1  "<IntkCamPhaseCmd>"
  Bus Selector4/34 -> Unit Conversion32/1  "<SpkAdv>"
  Bus Selector4/33 -> Unit Conversion31/1  "<InjPw>"
  Bus Selector4/31 -> Unit Conversion30/1  "<WgAreaPctCmd>"
  Bus Selector4/30 -> Unit Conversion26/1  "<ThrPosPctCmd>"
  Bus Selector4/29 -> Signal Specification54/1  "<TPCO2>"
  Bus Selector4/28 -> Signal Specification53/1  "<TPNOx>"
  Bus Selector4/27 -> Signal Specification52/1  "<TPCO>"
  Bus Selector4/26 -> Signal Specification51/1  "<TPHC>"
  Bus Selector4/25 -> Signal Specification41/1  "<BSFC>"
  Bus Selector4/24 -> Signal Specification50/1  "<IntercoolerTempOut>"
  Unit Conversion28/1 -> Signal Specification30/1
  Unit Conversion37/1 -> Signal Specification29/1
  Unit Conversion36/1 -> Signal Specification39/1
  Unit Conversion35/1 -> Signal Specification38/1
  Unit Conversion34/1 -> Signal Specification37/1
  Unit Conversion33/1 -> Signal Specification36/1
  Unit Conversion32/1 -> Signal Specification35/1
  Unit Conversion31/1 -> Signal Specification34/1
  Unit Conversion30/1 -> Signal Specification33/1
  Unit Conversion27/1 -> Signal Specification32/1
  Unit Conversion26/1 -> Signal Specification28/1
  Unit Conversion25/1 -> Signal Specification27/1
  Unit Conversion24/1 -> Signal Specification26/1
  Unit Conversion40/1 -> Signal Specification25/1
  Unit Conversion38/1 -> Signal Specification40/1
  Bus Selector4/23 -> Signal Specification49/1  "<EgrCoolerTempOut>"
  Bus Selector4/22 -> Signal Specification14/1  "<EgrMassFlwRate>"
  Bus Selector4/21 -> Bus Creator/24  "<EgrPct>"
  Bus Selector4/20 -> Signal Specification48/1  "<CompTempOut>"
  Bus Selector4/19 -> Signal Specification47/1  "<TurbTempOut>"
  Bus Selector4/18 -> Signal Specification46/1  "<CompPrsRatio>"
  Bus Selector4/17 -> Signal Specification45/1  "<TurbPrsRatio>"
  Bus Selector4/16 -> Unit Conversion18/1  "<TurboSpd>"
  Bus Selector4/15 -> Unit Conversion17/1  "<Afr>"
  Bus Selector4/14 -> Signal Specification58/1  "<ExhManGasTemp>"
  Bus Selector4/13 -> Signal Specification57/1  "<NormAirChrg>"
  Bus Selector4/12 -> Signal Specification56/1  "<IntkPortFlw>"
  Unit Conversion15/1 -> Signal Specification24/1
  Unit Conversion14/1 -> Signal Specification15/1
  Unit Conversion22/1 -> Signal Specification22/1
  Unit Conversion21/1 -> Signal Specification23/1
  Unit Conversion20/1 -> Signal Specification18/1
  Unit Conversion19/1 -> Signal Specification21/1
  Unit Conversion18/1 -> Signal Specification20/1
  Unit Conversion17/1 -> Signal Specification19/1
  Unit Conversion16/1 -> Signal Specification16/1
  Unit Conversion13/1 -> Signal Specification17/1
  Unit Conversion12/1 -> Signal Specification13/1
  Bus Selector4/11 -> Signal Specification/1  "<FuelFlw>"
  Bus Selector4/10 -> Unit Conversion10/1  "<TurboRackPos>"
  Bus Selector4/9 -> Unit Conversion9/1  "<EgrVlvAreaPct>"
  Bus Selector4/8 -> Unit Conversion8/1  "<ExhCamPhase>"
  Bus Selector4/7 -> Unit Conversion6/1  "<IntkCamPhase>"
  Bus Selector4/6 -> Gain2/1  "<WgAreaPct>"
  Unit Conversion11/1 -> Signal Specification12/1
  Unit Conversion10/1 -> Signal Specification11/1
  Unit Conversion9/1 -> Signal Specification10/1
  Unit Conversion8/1 -> Signal Specification9/1
  Gain2/1 -> Signal Specification8/1
  Unit Conversion6/1 -> Signal Specification7/1
  Bus Selector4/5 -> Gain1/1  "<ThrPosPct>"
  Gain1/1 -> Signal Specification6/1
  Bus Selector4/4 -> Unit Conversion4/1  "<Mat>"
  Unit Conversion4/1 -> Signal Specification5/1
  Unit Conversion3/1 -> Signal Specification4/1
  Unit Conversion2/1 -> Signal Specification3/1
  Unit Conversion1/1 -> Signal Specification2/1
  Unit Conversion/1 -> Signal Specification1/1
  Clock/1 -> Signal Specification31/1  "Time"
  Bus Selector3/2 -> Signal Specification42/1  "<SteadyStateFlag>"
  Bus Selector3/3 -> Unit Conversion1/1  "<TrqCmd>"
  Bus Selector3/1 -> Steady State Logging/Trigger  "<LogDataTrigger>"
  [EngSysResults] -> Bus Selector4/1
  [DynoResults] -> Bus Selector3/1
  Bus Selector4/1 -> Signal Specification55/1  "<EngTrq>"
  Bus Selector4/2 -> Unit Conversion2/1  "<EngSpdOut>"
  Bus Selector4/3 -> Unit Conversion3/1  "<Map>"
  Bus Creator/1 -> Unit Delay/1, Dynamic Logging/1(LogData)
  Unit Delay/1 -> Steady State Logging/1(LogData)
  Unit Conversion29/1 -> Signal Specification43/1
  Bus Selector4/32 -> Unit Conversion29/1  "<TurboRackPosCmd>"
  Signal Specification/1 -> Unit Conversion11/1
  Signal Specification45/1 -> Unit Conversion19/1
  Signal Specification46/1 -> Unit Conversion21/1
  Signal Specification47/1 -> Unit Conversion20/1
  Signal Specification48/1 -> Unit Conversion22/1
  Signal Specification14/1 -> Unit Conversion14/1
  Signal Specification49/1 -> Unit Conversion15/1
  Signal Specification50/1 -> Unit Conversion38/1
  Signal Specification51/1 -> Unit Conversion40/1
  Signal Specification52/1 -> Unit Conversion24/1
  Signal Specification53/1 -> Unit Conversion25/1
  Signal Specification54/1 -> Unit Conversion27/1
  Signal Specification55/1 -> Unit Conversion/1
  Signal Specification56/1 -> Unit Conversion13/1
  Signal Specification57/1 -> Unit Conversion12/1
  Signal Specification58/1 -> Unit Conversion16/1  "Exhaust manifold temperature (C)"

== system EngineDynamometer/Recalibrate CI Engine ==

== system EngineDynamometer/Recalibrate Engine ==

== system EngineDynamometer/Subsystem1 ==

== system EngineDynamometer/Subsystem3 ==

== system EngineDynamometer/Subsystem4 ==

== system EngineDynamometer/Subsystem5 ==

== system EngineDynamometer/Subsystem6 ==

== system EngineDynamometer/Dynamometer/Dynamometer Motor Controller ==
  EngPlnt : Inport
  DynoCtrl : Inport  Port=2
  DynoPlnt : Inport  Port=3
  Bus Creator : BusCreator  Inputs=2
  Bus Selector : BusSelector  OutputSignals=DynoCtrl.EngSpdCmd,DynoCtrl.FanFlwSpdCmd
  Terminator : Terminator
  Terminator1 : Terminator
  DynoMotorCtrl : Outport  VectorParamsAs1DForOutWhenUnconnected=off
  wires:
  DynoCtrl/1 -> Bus Selector/1
  EngPlnt/1 -> Terminator/1
  DynoPlnt/1 -> Terminator1/1
  Bus Selector/1 -> Bus Creator/1  "<EngSpdCmd>"
  Bus Creator/1 -> DynoMotorCtrl/1
  Bus Selector/2 -> Bus Creator/2  "<FanFlwSpdCmd>"

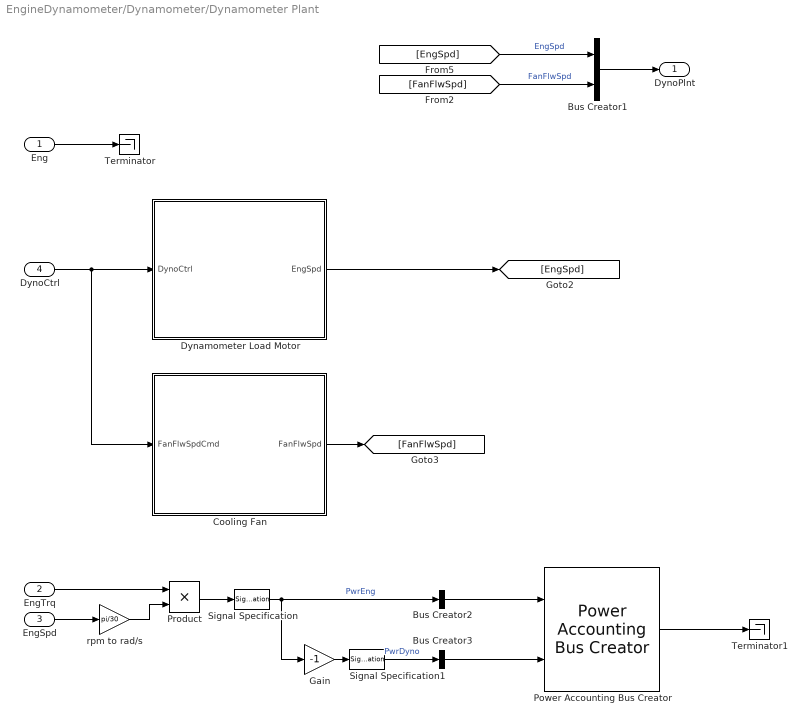
== system EngineDynamometer/Dynamometer/Dynamometer Plant ==
  Eng : Inport
  EngTrq : Inport  Port=2
  "EngSpd " : Inport  Port=3
  DynoCtrl : Inport  Port=4
  Bus Creator1 : BusCreator  Inputs=2
  Bus Creator2 : BusCreator  Inputs=1
  Bus Creator3 : BusCreator  Inputs=1
  Cooling Fan : Subsystem
  Dynamometer Load Motor : Subsystem
  Gain : Gain  Gain=-1
  Power Accounting Bus Creator : autolibpowerinfoutils/Power Accounting Bus Creator  AssctBlkSelPopup=Parent  RefBlkName='libraryname/blkname'  PwrTrnsfrdCheckBox=on  PwrNotTrnsfrdCheckBox=on  PwrStoredCheckBox=off  aMode=aMode
  Product : Product
  Signal Specification : SignalSpecification  Unit=W
  Signal Specification1 : SignalSpecification  Unit=W
  Terminator : Terminator
  Terminator1 : Terminator
  rpm to rad/s : Gain  Gain=pi/30
  DynoPlnt : Outport  VectorParamsAs1DForOutWhenUnconnected=off
  wires:
  Cooling Fan/1(FanFlwSpd) -> [FanFlwSpd]
  Dynamometer Load Motor/1(EngSpd) -> [EngSpd]
  Bus Creator1/1 -> DynoPlnt/1
  [EngSpd] -> Bus Creator1/1  "EngSpd"
  [FanFlwSpd] -> Bus Creator1/2  "FanFlwSpd"
  DynoCtrl/1 -> Cooling Fan/1(FanFlwSpdCmd), Dynamometer Load Motor/1(DynoCtrl)
  Eng/1 -> Terminator/1
  Bus Creator2/1 -> Power Accounting Bus Creator/1
  Signal Specification/1 -> Gain/1, Bus Creator2/1  "PwrEng"
  Bus Creator3/1 -> Power Accounting Bus Creator/2
  Power Accounting Bus Creator/1 -> Terminator1/1
  Gain/1 -> Signal Specification1/1
  Product/1 -> Signal Specification/1
  Signal Specification1/1 -> Bus Creator3/1  "PwrDyno"
  EngTrq/1 -> Product/1
  "EngSpd "/1 -> rpm to rad/s/1
  rpm to rad/s/1 -> Product/2
